simulink model "BitwiseNAND_int8"  (R2017b)
settings: Solver=FixedStepDiscrete  StartTime=0.0  StopTime=10.0  FixedStep=0.200000  RelTol=1e-3  EnableMultiTasking=on
model workspace (MAT data in the model file):
  already_pp = 0
  input_struct.time = [0; 0.2; 0.4; 0.6; 0.8; 1; 1.2; 1.4; 1.6; 1.8; 2; 2.2; 2.4; 2.6; 2.8; 3; 3.2; 3.4; 3.6; 3.8; 4; 4.2; 4.4; 4.6; 4.8; 5; 5.2; 5.4; 5.6; 5.8; 6; 6.2; 6.4; 6.6; 6.8; 7; 7.2; 7.4; 7.6; 7.8; 8; 8.2; 8.4; 8.6; 8.8; 9; 9.2; 9.4; 9.6; 9.8; 10; 10.2; 10.4; 10.6; 10.8; 11; 11.2; 11.4; 11.6; 11.8; 12; 12.2; 12.4; 12.6; 12.8; 13; 13.2; 13.4; 13.6; 13.8; 14; 14.2; 14.4; 14.6; 14.8; 15; 15.2; 15.4; 15.6; 15.8; 16; 16.2; 16.4; 16.6; 16.8; 17; 17.2; 17.4; 17.6; 17.8; 18; 18.2; 18.4; 18.6; 18.8; 19; 19.2; 19.4; 19.6; 19.8]
  input_struct.signals(1).name = 'In1'
  input_struct.signals(1).values = [-39; 48; 57; 7; -58; -23; 20; 62; -81; 54; 75; 67; 84; -18; 77; -4; -94; 92; 11; -43; -20; -36; 57; -99; 47; 21; 33; 68; -84; 39; -32; 51; -74; 44; -95; -19; 72; 65; -33; 31; -22; -12; 20; 98; -86; -29; -59; -19; -28; 58; 9; 42; 5; 17; -56; 37; -33; 38; 95; 41; 20; -66; 69; -2; -48; -59; 84; 55; 60; -75; -33; -32; -55; 100; -55; -46; -30; -27; 8; 10; -79; -3; -25; 7; 53; 14; -68; -61; -94; -2; -77; 11; -26; -17; -39; -26; -42; 75; 29; 51]
  input_struct.signals(1).dimensions = 1
  input_struct.signals(2).name = 'In2'
  input_struct.signals(2).values = [64; 62; -22; -92; -96; 75; 82; -37; 52; 30; 65; 71; -45; -77; 22; -69; -90; -25; 88; -60; -14; 1; -60; 26; -97; 64; -33; -65; -46; 36; -11; 80; -43; 12; -41; 89; 52; 15; -13; 62; 24; -28; -89; 50; 100; 17; -59; 54; 99; -35; 48; 51; 47; 35; 99; -12; 41; 74; -88; -63; -99; 73; 12; -83; -15; -90; -60; -71; -8; 61; -78; -23; 69; -13; 99; -27; 54; 34; -72; -81; 95; -71; -29; -66; 55; 51; -60; 78; -12; -12; 37; -78; 11; 94; 21; 31; 34; -13; 2; -54]
  input_struct.signals(2).dimensions = 1
  input_struct.signals(3).name = 'In3'
  input_struct.signals(3).values = [10; 18; 63; 64; -57; 41; 76; -47; 69; 61; -27; 47; 14; -37; -35; -21; -80; -46; -94; 33; 82; -25; -49; 75; 49; -47; -27; 55; 70; 34; -45; -57; 7; 28; -92; 88; 54; -21; 28; 13; -30; -57; 100; 41; 5; -17; -58; 61; -19; -80; 75; 23; 25; -41; 37; -15; 46; 27; 83; -47; -99; 46; 62; -25; -36; 79; -7; 85; 35; -75; -9; -33; 61; 5; -81; -9; 93; -11; -69; 17; 91; 70; -83; 72; 89; 99; 62; -51; -47; -79; -42; -68; 47; -12; 49; 100; 65; 15; -1; -54]
  input_struct.signals(3).dimensions = 1
  input_struct.signals(4).name = 'In4'
  input_struct.signals(4).values = [-70  -53  -92; 44  33  -75; 20  50  -8; 3  46  61; 69  63  -19; -43  48  51; 0  29  -32; -79  -81  -31; -35  100  23; 32  -16  89; 76  -85  -65; 53  48  -77; 63  100  -8; -4  10  96; -43  19  59; -9  -69  -69; -43  27  58; -29  9  44; 23  -43  -39; -17  32  -72; 85  99  99; -36  2  55; 50  -59  3; -59  27  -24; -39  37  -47; -46  -9  19; 39  -84  -79; -67  99  37; 6  -93  -59; -60  49  78; -69  17  24; 52  92  -93; 83  -20  70; -56  3  -72; -67  59  -54; 60  -21  -25; 22  -68  -60; 55  14  34; 11  20  -75; -41  64  68; 18  99  41; -68  -32  -41; -26  -100  51; 81  -88  67; -18  -7  -46; 66  98  5; 95  -93  -98; 12  -27  49; 37  -66  94; 9  74  96; 50  28  33; 29  78  -16; -71  53  -99; 68  -3  -28; -74  -87  38; 37  4  -19; 89  -19  -53; -9  16  92; -78  94  -51; -88  93  -93; 56  100  -48; -100  3  62; 21  45  60; -29  -71  -75; -21  -63  -75; -21  -53  -87; -16  84  66; 66  -84  17; 45  39  -32; 81  -63  52; 57  64  36; -35  -35  -46; -60  60  23; 31  64  -5; -79  -37  -60; 78  -60  18; 18  -68  72; 57  83  48; 19  42  70; -65  -76  3; -84  28  -32; 66  -71  -64; -70  -84  -84; -88  49  -7; 18  -62  -82; -7  -100  18; -8  -96  68; 82  -20  -92; -68  18  -23; 59  -91  6; 35  -100  30; 84  15  -79; 12  -30  52; -60  -68  -21; -49  25  -93; 25  10  -88; -25  70  -98; -28  -20  15; -95  -90  53; 54  100  -83]
  input_struct.signals(4).dimensions = 3
  input_struct.signals(5).name = 'In5'
  input_struct.signals(5).values = [-88  -76  -89; 28  42  40; 81  97  -14; -18  -12  -53; 57  -66  33; 1  -99  18; -48  -45  51; -24  -11  -35; -6  -92  47; 44  -89  -95; 16  -92  -79; -7  31  76; -48  -94  -34; 29  73  97; -93  -61  19; -88  -54  -48; 48  -82  -30; -96  84  -3; 30  -68  -45; 78  -29  61; 80  -84  -47; -41  19  -62; 63  -23  49; 14  -6  36; 87  98  40; 60  -68  -68; -45  89  -23; 100  -8  27; 46  89  -70; -43  -34  -68; 18  78  63; 50  -94  65; -10  43  76; -92  72  -77; 92  -42  28; -3  24  13; -84  97  72; -90  2  50; 26  63  -94; -39  38  71; 48  -93  -6; 13  -78  -3; 43  98  3; 29  -48  -22; -39  -86  -23; 9  -97  -59; 60  0  -79; 36  -58  43; 95  61  -96; 32  14  100; -51  -34  -85; -10  3  -22; -50  -17  -34; 52  9  31; 4  94  -1; -79  -85  -96; 37  -91  -92; 33  -45  -19; 82  24  -6; -2  -21  91; -7  42  -42; 33  -23  32; 88  -75  34; -35  -29  -98; -96  68  43; 55  44  -6; -83  13  -83; 7  -44  -9; 60  17  -26; 10  -22  90; 61  -66  -51; -37  -96  59; -21  83  81; -6  70  82; -47  75  -55; 56  51  -33; -1  23  -97; 26  -60  -17; 2  -49  64; 69  -99  69; 61  -32  -84; -1  50  94; 74  -44  -70; -1  -100  55; 93  -94  0; -86  38  45; -25  -46  57; 18  -81  91; -57  -24  22; 35  27  -39; 34  -32  79; 51  26  -29; 57  31  -77; 23  84  -28; 62  44  -13; -42  -78  42; -48  37  79; -88  -53  -78; 45  76  75; -11  26  -83]
  input_struct.signals(5).dimensions = 3
  input_struct.signals(6).name = 'In6'
  input_struct.signals(6).values = [-57  -90  85; -99  95  12; -21  -98  88; 35  2  -100; 58  -71  -14; 4  8  21; 11  79  58; -1  -9  95; 88  -67  70; 79  -25  100; 17  -47  30; 3  98  -69; -30  80  -95; -67  26  90; 30  -38  -80; -70  12  12; -74  55  53; -80  -84  8; 64  46  -6; -79  -10  42; -28  -71  -45; 52  -83  -6; 74  80  73; -85  -9  18; 13  78  98; -31  -19  89; -66  10  90; 66  -83  13; 19  56  -98; 63  -75  -38; -32  -77  75; 81  13  -67; -77  94  73; 18  -15  32; 29  0  -79; -88  58  95; 63  17  -59; 92  -6  9; 52  -5  -97; -2  -32  16; 19  26  -13; -26  -75  -62; -71  12  87; -42  84  62; 28  -33  34; -10  -35  -40; 74  15  -89; 39  38  -86; 21  25  35; -22  86  9; -6  -34  -3; -42  -17  13; 95  -33  62; -84  -53  59; -14  -20  -78; -84  91  0; 71  -62  -86; 77  22  74; -55  -69  76; -4  -49  79; 28  60  28; -19  -54  40; -82  -26  -21; 40  -37  56; 57  78  -44; 37  -95  -75; 40  26  72; -34  -54  98; 35  43  31; 64  -85  -90; 77  95  66; 57  -19  84; -7  66  -83; 58  -43  86; -45  -97  78; -87  15  -52; 97  -89  -20; -7  21  -80; -70  24  92; -26  57  -65; -19  9  2; 12  -5  -15; 59  -34  27; -47  -44  9; -28  70  -75; -76  -58  -1; 3  -73  0; 59  13  -15; 81  38  21; -72  -28  -83; -55  38  -57; -39  -31  -28; 1  66  -54; -56  32  -72; -25  -29  44; -24  -84  -43; 47  20  14; 62  80  -80; 50  91  90; -60  -14  -27]
  input_struct.signals(6).dimensions = 3
settings Model: Creator=hbourbou  LastModifiedBy=hbourbou
settings OptimizationCC: LifeSpan=inf
settings DebuggingCC: AlgebraicLoopMsg=error  ArtificialAlgebraicLoopMsg=error  SFExecutionAtInitializationDiag=none
settings HardwareCC: ProdBitPerSizeT=32  ProdBitPerPtrDiffT=32  ProdWordSize=32  ProdHWDeviceType=Specified
settings CodeAppCC: StateflowObjectComments=on

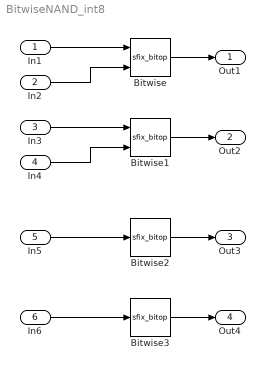
== system BitwiseNAND_int8 ==
  In1 : Inport  OutDataTypeStr=int8  PortDimensions=1
  In2 : Inport  Port=2  OutDataTypeStr=int8  PortDimensions=1
  In3 : Inport  Port=3  OutDataTypeStr=int8  PortDimensions=1
  In4 : Inport  Port=4  OutDataTypeStr=int8  PortDimensions=3
  In5 : Inport  Port=5  OutDataTypeStr=int8  PortDimensions=3
  In6 : Inport  Port=6  OutDataTypeStr=int8  PortDimensions=3
  Bitwise : S-Function  FunctionName=sfix_bitop  Parameters=UseBitMask,NumInputPorts,BitMask,BitMaskRealWorld,logicop  SFunctionDeploymentMode=off  EnableBusSupport=off  mask(Bitwise Operator){logicop=NAND, UseBitMask=off, NumInputPorts=2, BitMask=bin2dec('11011001'), BitMaskRealWorld=Stored Integer}
      mask prompts: logicop "Simulink:masks:Operator_MP"; UseBitMask "Simulink:masks:UseBitMask_MP"; NumInputPorts "Simulink:masks:NumberOfInputPorts_MP"; BitMask "Simulink:masks:BitMask_MP"; BitMaskRealWorld "Simulink:masks:TreatMaskAs_MP"
      mask help: Simulink:masks:BitwiseOperator_MD
      mask init:
      | str = '';
      | if UseBitMask
      |   [m,n] = size(BitMask);
      |   if ischar(BitMask)
      |     len = m;
      |     n = 1;
      |   else
      |     len = m * n;
      |   end
      |   internalBitMask = zeros(m,n);
      |   if isnumeric(BitMask)
      |     if ~isreal(BitMask)
      |       error(DAStudio.message('Simulink:blocks:BitMaskNotComplex'));
      |     end
      |     for i=1:len,
      |       internalBitMask(i) = BitMask(i);
      |     end
      |   elseif ischar(BitMask)
      |     for i=1:m,
      |       internalBitMask(i) = hex2dec(BitMask(i,:));
      |     end
      |   elseif iscell(BitMask)
      |     for i=1:len,
      |       if isnumeric( BitMask{i} )
      |         internalBitMask(i) = BitMask{i};
      |       elseif ischar( BitMask{i} )
      |         internalBitMask(i) = hex2dec(BitMask{i});
      |       else
      |         errordlg(['Data type is not supported at cell item ', num2str(i) ]);
      |       end
      |     end
      |   end
      |   BitMask = internalBitMask;
      |   for i=1:len
      |     if BitMask(i) > (2^52)-1
      |       error(DAStudio.message('Simulink:blocks:BitMaskWordLengthTooLarge')); 
      |     end
      |   end 
      |   if len == 1
      |      if BitMaskRealWorld == 1 || BitMask(1) < 0
      |        str=num2str(BitMask(1));
      |      else
      |        str=['0x',dec2hex(floor(BitMask(1)))];
      |      end
      |   else
      |      str='Masks';
      |   end
      | else
      |   BitMask = 0;
      |   str='';
      | end
      mask TypeOptions logicop: Simulink:masks:AND | Simulink:masks:OR | Simulink:masks:NAND | Simulink:masks:NOR | Simulink:masks:XOR | Simulink:masks:NOT
      mask Callback logicop: fixptdialog(gcbh)
      mask Callback UseBitMask: fixptdialog(gcbh)
      mask TypeOptions BitMaskRealWorld: Simulink:masks:RealWorldValue | Simulink:masks:StoredInteger
      mask Display: fprintf(['Bitwise\n',logicop,'\n',str])
  Bitwise1 : S-Function  FunctionName=sfix_bitop  Parameters=UseBitMask,NumInputPorts,BitMask,BitMaskRealWorld,logicop  SFunctionDeploymentMode=off  EnableBusSupport=off  mask(Bitwise Operator){logicop=NAND, UseBitMask=off, NumInputPorts=2, BitMask=bin2dec('11011001'), BitMaskRealWorld=Stored Integer}
      mask prompts: logicop "Simulink:masks:Operator_MP"; UseBitMask "Simulink:masks:UseBitMask_MP"; NumInputPorts "Simulink:masks:NumberOfInputPorts_MP"; BitMask "Simulink:masks:BitMask_MP"; BitMaskRealWorld "Simulink:masks:TreatMaskAs_MP"
      mask help: Simulink:masks:BitwiseOperator_MD
      mask init: same as BitwiseNAND_int8/Bitwise
      mask TypeOptions logicop: Simulink:masks:AND | Simulink:masks:OR | Simulink:masks:NAND | Simulink:masks:NOR | Simulink:masks:XOR | Simulink:masks:NOT
      mask Callback logicop: fixptdialog(gcbh)
      mask Callback UseBitMask: fixptdialog(gcbh)
      mask TypeOptions BitMaskRealWorld: Simulink:masks:RealWorldValue | Simulink:masks:StoredInteger
      mask Display: fprintf(['Bitwise\n',logicop,'\n',str])
  Bitwise2 : S-Function  FunctionName=sfix_bitop  Parameters=UseBitMask,NumInputPorts,BitMask,BitMaskRealWorld,logicop  SFunctionDeploymentMode=off  EnableBusSupport=off  mask(Bitwise Operator){logicop=NAND, UseBitMask=on, NumInputPorts=1, BitMask=bin2dec('11011001'), BitMaskRealWorld=Stored Integer}
      mask prompts: logicop "Simulink:masks:Operator_MP"; UseBitMask "Simulink:masks:UseBitMask_MP"; NumInputPorts "Simulink:masks:NumberOfInputPorts_MP"; BitMask "Simulink:masks:BitMask_MP"; BitMaskRealWorld "Simulink:masks:TreatMaskAs_MP"
      mask help: Simulink:masks:BitwiseOperator_MD
      mask init: same as BitwiseNAND_int8/Bitwise
      mask TypeOptions logicop: Simulink:masks:AND | Simulink:masks:OR | Simulink:masks:NAND | Simulink:masks:NOR | Simulink:masks:XOR | Simulink:masks:NOT
      mask Callback logicop: fixptdialog(gcbh)
      mask Callback UseBitMask: fixptdialog(gcbh)
      mask TypeOptions BitMaskRealWorld: Simulink:masks:RealWorldValue | Simulink:masks:StoredInteger
      mask Display: fprintf(['Bitwise\n',logicop,'\n',str])
  Bitwise3 : S-Function  FunctionName=sfix_bitop  Parameters=UseBitMask,NumInputPorts,BitMask,BitMaskRealWorld,logicop  SFunctionDeploymentMode=off  EnableBusSupport=off  mask(Bitwise Operator){logicop=NAND, UseBitMask=off, NumInputPorts=1, BitMask=bin2dec('11011001'), BitMaskRealWorld=Stored Integer}
      mask prompts: logicop "Simulink:masks:Operator_MP"; UseBitMask "Simulink:masks:UseBitMask_MP"; NumInputPorts "Simulink:masks:NumberOfInputPorts_MP"; BitMask "Simulink:masks:BitMask_MP"; BitMaskRealWorld "Simulink:masks:TreatMaskAs_MP"
      mask help: Simulink:masks:BitwiseOperator_MD
      mask init: same as BitwiseNAND_int8/Bitwise
      mask TypeOptions logicop: Simulink:masks:AND | Simulink:masks:OR | Simulink:masks:NAND | Simulink:masks:NOR | Simulink:masks:XOR | Simulink:masks:NOT
      mask Callback logicop: fixptdialog(gcbh)
      mask Callback UseBitMask: fixptdialog(gcbh)
      mask TypeOptions BitMaskRealWorld: Simulink:masks:RealWorldValue | Simulink:masks:StoredInteger
      mask Display: fprintf(['Bitwise\n',logicop,'\n',str])
  Out1 : Outport
  Out2 : Outport  Port=2
  Out3 : Outport  Port=3
  Out4 : Outport  Port=4
  wires:
  In1/1 -> Bitwise/1
  In2/1 -> Bitwise/2
  Bitwise/1 -> Out1/1
  Bitwise1/1 -> Out2/1
  In3/1 -> Bitwise1/1
  In4/1 -> Bitwise1/2
  In5/1 -> Bitwise2/1
  Bitwise2/1 -> Out3/1
  Bitwise3/1 -> Out4/1
  In6/1 -> Bitwise3/1
